simulink model "decision_buffer"  (R2021a)
settings: Solver=FixedStepAuto  StartTime=0.0  StopTime=inf  FixedStep=0.001  RelTol=1e-3
settings Model: OrderedModelArguments=off  Creator=Ruixuan
settings SolverCC: ConcurrentTasks=on  PositivePriorityOrder=on  AutoInsertRateTranBlk=on  InsertRTBMode=Never (minimum delay)
settings OptimizationCC: BlockReduction=off  DefaultParameterBehavior=Inlined  OptimizeBlockIOStorage=off
settings DebuggingCC: TasksWithSamePriorityMsg=none
settings HardwareCC: ProdBitPerLong=64  ProdLongLongMode=on  ProdHWDeviceType=Intel->x86-64 (Linux 64)
settings RTWCC: Description=Simulink Real-Time  SystemTargetFile=slrealtime.tlc  TemplateMakefile=slrealtime_default_tmf  Toolchain=Simulink Real-Time Toolchain  BuildConfiguration=Faster Runs  CodeExecutionProfiling=on  TargetLang=C++

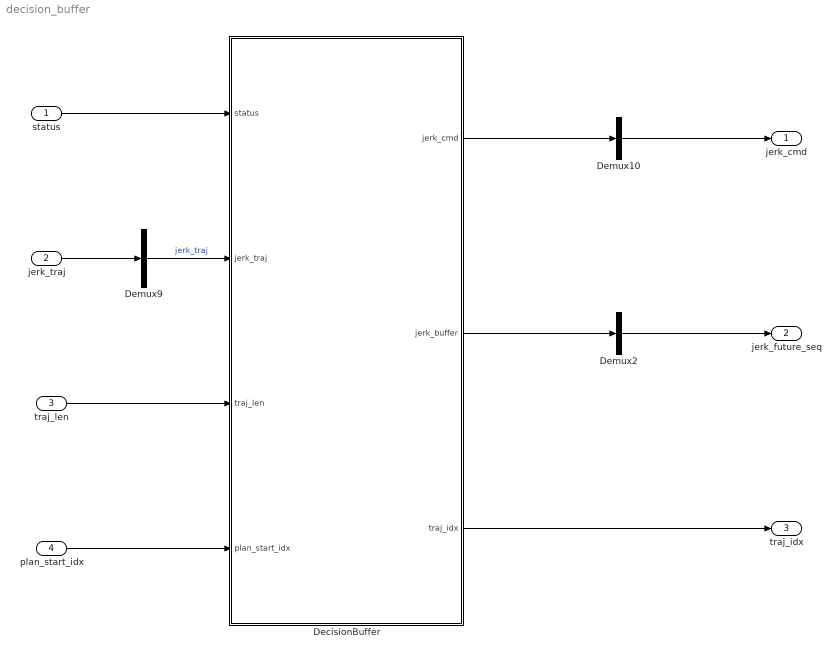
== system decision_buffer ==
  status : Inport
  jerk_traj : Inport  Port=2
  traj_len : Inport  Port=3
  plan_start_idx : Inport  Port=4
  DecisionBuffer : MATLAB Function  TreatAsAtomicUnit=on
  Demux10 : Demux  Outputs=[9]
  Demux2 : Demux  Outputs=[30]
  Demux9 : Demux  Outputs=[11250]
  jerk_cmd : Outport  VectorParamsAs1DForOutWhenUnconnected=off
  jerk_future_seq : Outport  Port=2  VectorParamsAs1DForOutWhenUnconnected=off
  traj_idx : Outport  Port=3  VectorParamsAs1DForOutWhenUnconnected=off
  wires:
  DecisionBuffer/2(jerk_buffer) -> Demux2/1
  status/1 -> DecisionBuffer/1(status)
  traj_len/1 -> DecisionBuffer/3(traj_len)
  Demux2/1 -> jerk_future_seq/1
  plan_start_idx/1 -> DecisionBuffer/4(plan_start_idx)
  DecisionBuffer/3(traj_idx) -> traj_idx/1
  jerk_traj/1 -> Demux9/1
  Demux9/1 -> DecisionBuffer/2(jerk_traj)  "jerk_traj"
  Demux10/1 -> jerk_cmd/1
  DecisionBuffer/1(jerk_cmd) -> Demux10/1

== matlab function decision_buffer/DecisionBuffer ==
  data: jerk_cmd output; status input; jerk_traj input; traj_len input; plan_start_idx input; jerk_buffer output; traj_idx output
% This function implements the buffer that stores and organizes the nominal jerk control command.
% Copyright (C) 2022  
% 
% Authors:
% Ruixuan Liu: ruixuanl@andrew.cmu.edu
% Rui Chen: ruic3@andrew.cmu.edu
% Changliu Liu : cliu6@andrew.cmu.edu
% 
% This program is free software; you can redistribute it and/or
% modify it under the terms of the GNU General Public License
% as published by the Free Software Foundation; either version 2
% of the License, or (at your option) any later version.
% 
% This program is distributed in the hope that it will be useful,
% but WITHOUT ANY WARRANTY; without even the implied warranty of
% MERCHANTABILITY or FITNESS FOR A PARTICULAR PURPOSE.  See the
% GNU General Public License for more details.
% 
% You should have received a copy of the GNU General Public License
% along with this program; if not, write to the Free Software
% Foundation, Inc., 51 Franklin Street, Fifth Floor, Boston, MA  02110-1301, USA.

function [jerk_cmd, jerk_buffer, traj_idx]  = DecisionBuffer(status,jerk_traj,traj_len,plan_start_idx)

    persistent m_jerk_buffer m_traj_horizon m_traj_T m_status m_T m_switch;
    jerk_cmd = zeros(9,1);
    jerk_buffer = zeros(5*6,1);

    if isempty(m_status)
       [m_jerk_buffer, m_traj_horizon, m_traj_T, m_T, m_status, m_switch]=reset();
    end
    
    % Have incoming traj
    if status && m_switch==0
        m_switch = 1;
        if m_traj_T == 0 % No ongoing trajectory
            m_traj_horizon = traj_len;
            m_traj_T = 0;
            m_T = 0;
            m_status = 1;
            m_jerk_buffer(1:traj_len*6) = jerk_traj(1:traj_len*6);
        else
            m_jerk_buffer((plan_start_idx)*6+1:(plan_start_idx+traj_len)*6) = jerk_traj(1:traj_len*6);
            m_traj_horizon = traj_len + plan_start_idx - m_traj_T + 1;
            %original code, but error
            % m_jerk_buffer(1:m_traj_horizon*6) = m_jerk_buffer((m_traj_T-1)*6+1:(plan_start_idx+traj_len+1)*6);
            m_jerk_buffer(1:m_traj_horizon*6) = m_jerk_buffer((m_traj_T-1)*6+1:(plan_start_idx+traj_len)*6);
            m_traj_T = 1;
            m_status = 1;
        end
    end
        
    % Have no valid pos in buffer
    if ~m_status
        m_T = 0;
        m_traj_T = 0;
        traj_idx = 0;
        return;
    end
    m_T = m_T + 1;
    if m_traj_T > m_traj_horizon
        [m_jerk_buffer, m_traj_horizon, m_traj_T, m_T, m_status, m_switch]=reset();
    end
    if(mod(m_T, 8) == 1)
        m_traj_T = m_traj_T + 1;
        if ~status
            m_switch = 0;
        end
    end
    if m_traj_T == 0
        jerk_cmd(1:6) = m_jerk_buffer(1:6);    %zeros(1, 6) m_jerk_buffer(1:6)
    else
        jerk_cmd(1:6) = m_jerk_buffer((m_traj_T-1)*6+1:(m_traj_T-1)*6+6);
    end
%     jerk_cmd(1:6) = m_jerk_buffer((m_traj_T-1)*6+1:(m_traj_T-1)*6+6);
    jerk_cmd(7) = m_traj_T;
    jerk_cmd(8) = m_traj_horizon;
    jerk_cmd(9) = m_status;
    for i=1:5
        jerk_buffer((i-1)*6+1:i*6) = m_jerk_buffer((m_traj_T+i-1)*6+1:(m_traj_T+i-1)*6+6);
    end
    
    traj_idx = m_traj_T;
    
    
function [m_jerk_buffer, m_traj_horizon, m_traj_T, m_T, m_status, m_switch]=reset()
    max_traj_len = 1875;
    m_jerk_buffer = zeros(max_traj_len*6, 1);
    m_traj_horizon = 0;
    m_traj_T = 0;
    m_status = 0;
    m_T = 0;
    m_switch = 0;
